simulink model "vcv_model"  (R2024b)
settings: Solver=VariableStepAuto  StartTime=0.0  StopTime=60.0  RelTol=1e-3
values from neighbouring files (symbols this model uses):
  C = 0.0965    [vcv.m]
  R = 4    [vcv.m]
libraries: slpidlib x2
settings Model: Creator=Neuer Benutzer  LastModifiedBy=Neuer Benutzer

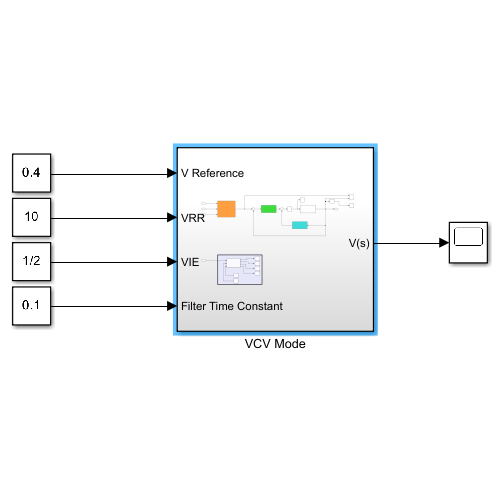
[thumbnail: Simulink's stored preview of the top-level diagram]
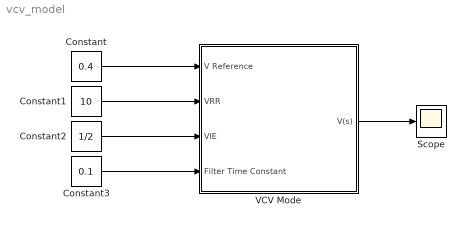
== system vcv_model ==
  Constant : Constant  Value=0.4
  Constant1 : Constant  Value=10
  Constant2 : Constant  Value=1/2
  Constant3 : Constant  Value=0.1
  Scope : Scope
  VCV Mode : Subsystem
  wires:
  Constant/1 -> VCV Mode/1(V Reference)
  Constant1/1 -> VCV Mode/2("VRR ")
  Constant2/1 -> VCV Mode/3(VIE)
  Constant3/1 -> VCV Mode/4("Filter Time Constant ")
  VCV Mode/1(V(s)) -> Scope/1

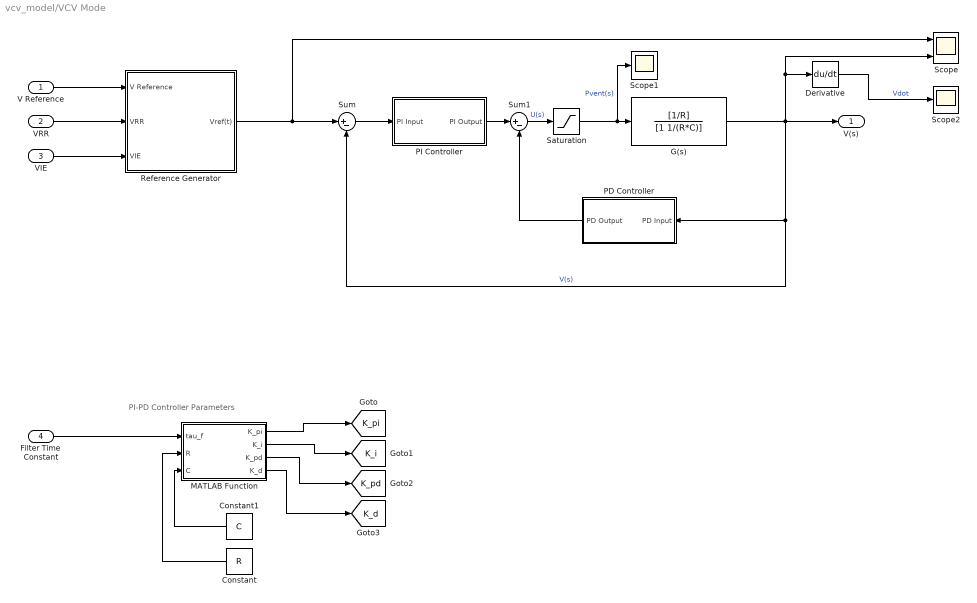
== system vcv_model/VCV Mode ==
  note: PI-PD Controller Parameters
  V Reference : Inport
  "VRR " : Inport  Port=2
  VIE : Inport  Port=3
  "Filter Time Constant " : Inport  Port=4
  Constant : Constant  Value=R
  Constant1 : Constant  Value=C
  Derivative : Derivative
  G(s) : TransferFcn  Numerator=[1/R]  Denominator=[1 1/(R*C)]
  MATLAB Function : MATLAB Function  TreatAsAtomicUnit=on
  PD Controller : Subsystem
  PI Controller : Subsystem
  Reference Generator : Subsystem
  Saturation : Saturate  UpperLimit=30  LowerLimit=0
  Scope : Scope  NumInputPorts=2
  Scope1 : Scope
  Scope2 : Scope
  Sum : Sum  Inputs=|+-
  Sum1 : Sum  Inputs=|+-
  V(s) : Outport
  tag scope: K_d=global, K_i=global, K_pd=global, K_pi=global
  wires:
  G(s)/1 -> Derivative/1, Scope/2, V(s)/1, Sum/2, PD Controller/1(PD Input)  "V(s)"
  Reference Generator/1(Vref(t)) -> Sum/1, Scope/1
  Saturation/1 -> Scope1/1, G(s)/1  "Pvent(s)"
  PD Controller/1(PD Output) -> Sum1/2
  "Filter Time Constant "/1 -> MATLAB Function/1(tau_f)
  "VRR "/1 -> Reference Generator/2("VRR ")
  V Reference/1 -> Reference Generator/1(V Reference)
  VIE/1 -> Reference Generator/3(VIE)
  PI Controller/1(PI Output) -> Sum1/1
  Sum/1 -> PI Controller/1(PI Input)
  Sum1/1 -> Saturation/1  "U(s)"
  MATLAB Function/1(K_pi) -> [K_pi]
  MATLAB Function/2(K_i) -> [K_i]
  MATLAB Function/3(K_pd) -> [K_pd]
  MATLAB Function/4(K_d) -> [K_d]
  Constant/1 -> MATLAB Function/2(R)
  Constant1/1 -> MATLAB Function/3(C)
  Derivative/1 -> Scope2/1  "Vdot"

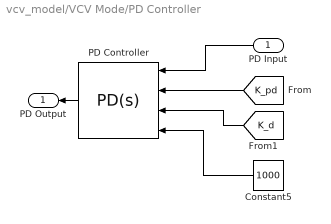
== system vcv_model/VCV Mode/PD Controller ==
  PD Input : Inport
  Constant5 : Constant  Value=1000
  PD Controller : slpidlib/PID Controller  Controller=PD  Form=Parallel  TimeDomain=Continuous-time  UseExternalTs=off  SampleTime=-1  IntegratorMethod=Forward Euler  FilterMethod=Forward Euler  ControllerParametersSource=external  P=1  I=1  UseKiTs=off  D=0  UseExternalDerivativeSource=off  N=100  UseFilter=on  TunerSelectOption=Transfer Function Based (PID Tuner App)  InitialConditionSource=internal  InitialConditionForIntegrator=0  InitialConditionForFilter=0  DifferentiatorICPrevScaledInput=0  ExternalReset=none  TrackingMode=off  Kt=1  LimitOutput=off  SatLimitsSource=internal  UpperSaturationLimit=30  LowerSaturationLimit=0  LinearizeAsGain=on  AntiWindupMode=none  Kb=1  LimitIntegrator=off  UpperIntegratorSaturationLimit=inf  LowerIntegratorSaturationLimit=-inf  POutMin=[]  POutMax=[]  IOutMin=[]  IOutMax=[]  DOutMin=[]  DOutMax=[]  NOutMin=[]  NOutMax=[]  SumOutMin=[]  SumOutMax=[]  SaturationOutMin=[]  SaturationOutMax=[]  PParamMin=[]  PParamMax=[]  IParamMin=[]  IParamMax=[]  DParamMin=[]  DParamMax=[]  NParamMin=[]  NParamMax=[]  KbParamMin=[]  KbParamMax=[]  KtParamMin=[]  KtParamMax=[]  KbOutMin=[]  KbOutMax=[]  KtOutMin=[]  KtOutMax=[]  IntegratorOutMin=[]  IntegratorOutMax=[]  FilterOutMin=[]  FilterOutMax=[]  SumI1OutMin=[]  SumI1OutMax=[]  SumI2OutMin=[]  SumI2OutMax=[]  SumI3OutMin=[]  SumI3OutMax=[]  SumI4OutMin=[]  SumI4OutMax=[]  SumDOutMin=[]  SumDOutMax=[]  DifferentiatorOutMin=[]  DifferentiatorOutMax=[]  FilterDiffOutCoefMin=[]  FilterDiffOutCoefMax=[]  ReciprocalOutMin=[]  ReciprocalOutMax=[]  SumDenOutMin=[]  SumDenOutMax=[]  SumNumOutMin=[]  SumNumOutMax=[]  DivideOutMin=[]  DivideOutMax=[]  UdiffTsProdOutMin=[]  UdiffTsProdOutMax=[]  NTsProdOutMin=[]  NTsProdOutMax=[]  UintegralTsProdOutMin=[]  UintegralTsProdOutMax=[]  UngainTsProdOutMin=[]  UngainTsProdOutMax=[]  ClampingZeroOutDataTypeStr=Inherit: Inherit via back propagation  ClampingZeroOutMin=[]  ClampingZeroOutMax=[]  FilterDenConstantOutDataTypeStr=Inherit: Inherit via back propagation  FilterDenConstantOutMin=[]  FilterDenConstantOutMax=[]  PCopyOutDataTypeStr=Inherit: Inherit via back propagation  PCopyOutMin=[]  PCopyOutMax=[]  NCopyOutDataTypeStr=Inherit: Inherit via back propagation  NCopyOutMin=[]  NCopyOutMax=[]  IntegratorContinuousStateAttributes=''  IntegratorStateMustResolveToSignalObject=off  IntegratorRTWStateStorageClass=Auto  FilterContinuousStateAttributes=''  FilterStateMustResolveToSignalObject=off  FilterRTWStateStorageClass=Auto  ParallelPVariant=ExternalParameters  IdealPVariant=Disabled  IVariant=Disabled  DVariant=ExternalParameters  IntegratorVariant=Disabled  SatVariant=Disabled  AWVariant=Disabled  PCopyVariant=Disabled  TRVariant=Disabled  FdbkBlocksVariant=Forward  IdealPFdbkVariant=Disabled  SatFdbkVariant=Disabled  DerivativeFilterVariant=ContFilter  NVariant=ExternalParameters  NCopyVariant=Disabled  FilterICVariant=InternalICsFilter  IntegratorICVariant=Disabled  ExternalResetVariant=Disabled  TRSumVariant=Passthrough  SumFdbkVariant=Disabled  SumVariant=Sum_PD  TsampFilterVariant=InternalTs  TsampNgainVariant=Passthrough  TsampIntegralVariant=Disabled_SignalSpec  ExternalSaturationOutDataTypeStr=Inherit: Same as second input  DerivativeSourceVariant=ErrorSignal  PreIntVariant=InternalPreInt
      settings: LibrarySourceBlock=cstblocks/Linear Parameter Varying/Varying PID Controller
  PD Output : Outport
  wires:
  PD Controller/1 -> PD Output/1
  Constant5/1 -> PD Controller/4
  PD Input/1 -> PD Controller/1
  [K_pd] -> PD Controller/2
  [K_d] -> PD Controller/3

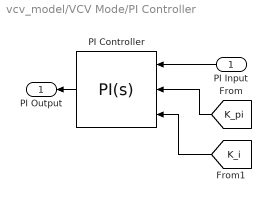
== system vcv_model/VCV Mode/PI Controller ==
  PI Input : Inport
  PI Controller : slpidlib/PID Controller  Controller=PI  Form=Parallel  TimeDomain=Continuous-time  UseExternalTs=off  SampleTime=-1  IntegratorMethod=Forward Euler  FilterMethod=Forward Euler  ControllerParametersSource=external  P=1  I=1  UseKiTs=off  D=0  UseExternalDerivativeSource=off  N=100  UseFilter=on  TunerSelectOption=Transfer Function Based (PID Tuner App)  InitialConditionSource=internal  InitialConditionForIntegrator=0  InitialConditionForFilter=0  DifferentiatorICPrevScaledInput=0  ExternalReset=none  TrackingMode=off  Kt=1  LimitOutput=off  SatLimitsSource=internal  UpperSaturationLimit=30  LowerSaturationLimit=0  LinearizeAsGain=on  AntiWindupMode=none  Kb=1  LimitIntegrator=off  UpperIntegratorSaturationLimit=inf  LowerIntegratorSaturationLimit=-inf  POutMin=[]  POutMax=[]  IOutMin=[]  IOutMax=[]  DOutMin=[]  DOutMax=[]  NOutMin=[]  NOutMax=[]  SumOutMin=[]  SumOutMax=[]  SaturationOutMin=[]  SaturationOutMax=[]  PParamMin=[]  PParamMax=[]  IParamMin=[]  IParamMax=[]  DParamMin=[]  DParamMax=[]  NParamMin=[]  NParamMax=[]  KbParamMin=[]  KbParamMax=[]  KtParamMin=[]  KtParamMax=[]  KbOutMin=[]  KbOutMax=[]  KtOutMin=[]  KtOutMax=[]  IntegratorOutMin=[]  IntegratorOutMax=[]  FilterOutMin=[]  FilterOutMax=[]  SumI1OutMin=[]  SumI1OutMax=[]  SumI2OutMin=[]  SumI2OutMax=[]  SumI3OutMin=[]  SumI3OutMax=[]  SumI4OutMin=[]  SumI4OutMax=[]  SumDOutMin=[]  SumDOutMax=[]  DifferentiatorOutMin=[]  DifferentiatorOutMax=[]  FilterDiffOutCoefMin=[]  FilterDiffOutCoefMax=[]  ReciprocalOutMin=[]  ReciprocalOutMax=[]  SumDenOutMin=[]  SumDenOutMax=[]  SumNumOutMin=[]  SumNumOutMax=[]  DivideOutMin=[]  DivideOutMax=[]  UdiffTsProdOutMin=[]  UdiffTsProdOutMax=[]  NTsProdOutMin=[]  NTsProdOutMax=[]  UintegralTsProdOutMin=[]  UintegralTsProdOutMax=[]  UngainTsProdOutMin=[]  UngainTsProdOutMax=[]  ClampingZeroOutDataTypeStr=Inherit: Inherit via back propagation  ClampingZeroOutMin=[]  ClampingZeroOutMax=[]  FilterDenConstantOutDataTypeStr=Inherit: Inherit via back propagation  FilterDenConstantOutMin=[]  FilterDenConstantOutMax=[]  PCopyOutDataTypeStr=Inherit: Inherit via back propagation  PCopyOutMin=[]  PCopyOutMax=[]  NCopyOutDataTypeStr=Inherit: Inherit via back propagation  NCopyOutMin=[]  NCopyOutMax=[]  IntegratorContinuousStateAttributes=''  IntegratorStateMustResolveToSignalObject=off  IntegratorRTWStateStorageClass=Auto  FilterContinuousStateAttributes=''  FilterStateMustResolveToSignalObject=off  FilterRTWStateStorageClass=Auto  ParallelPVariant=ExternalParameters  IdealPVariant=Disabled  IVariant=ExternalParameters  DVariant=Disabled  IntegratorVariant=Continuous  SatVariant=Disabled  AWVariant=Passthrough  PCopyVariant=Disabled  TRVariant=Disabled  FdbkBlocksVariant=Forward  IdealPFdbkVariant=Disabled  SatFdbkVariant=Disabled  DerivativeFilterVariant=Disabled  NVariant=Disabled  NCopyVariant=Disabled_SignalSpec  FilterICVariant=Disabled  IntegratorICVariant=InternalICs  ExternalResetVariant=Disabled  TRSumVariant=Passthrough  SumFdbkVariant=Disabled  SumVariant=Sum_PI  TsampFilterVariant=InternalTs  TsampNgainVariant=Passthrough  TsampIntegralVariant=Disabled_SignalSpec  ExternalSaturationOutDataTypeStr=Inherit: Same as second input  DerivativeSourceVariant=Disabled  PreIntVariant=InternalPreInt
      settings: LibrarySourceBlock=cstblocks/Linear Parameter Varying/Varying PID Controller
  PI Output : Outport
  wires:
  PI Input/1 -> PI Controller/1
  PI Controller/1 -> PI Output/1
  [K_pi] -> PI Controller/2
  [K_i] -> PI Controller/3

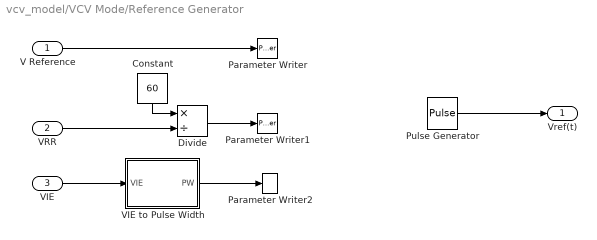
== system vcv_model/VCV Mode/Reference Generator ==
  V Reference : Inport
  "VRR " : Inport  Port=2
  VIE : Inport  Port=3
  Constant : Constant  Value=60
  Divide : Product  Inputs=*/
  Parameter Writer : ParameterWriter  ParameterOwnerBlock=../Pulse Generator  ParameterName=Amplitude  ParameterInternalName=Amplitude
  Parameter Writer1 : ParameterWriter  ParameterOwnerBlock=../Pulse Generator  ParameterName=Period  ParameterInternalName=Period
  Parameter Writer2 : ParameterWriter  ParameterOwnerBlock=../Pulse Generator  ParameterName=PulseWidth  ParameterInternalName=PulseWidth
  Pulse Generator : DiscretePulseGenerator  PulseType=Time based  Amplitude=10  Period=1  PulseWidth=70
  VIE to Pulse Width : MATLAB Function  TreatAsAtomicUnit=on
  Vref(t) : Outport
  wires:
  Constant/1 -> Divide/1
  Pulse Generator/1 -> Vref(t)/1
  "VRR "/1 -> Divide/2
  Divide/1 -> Parameter Writer1/1
  VIE/1 -> VIE to Pulse Width/1(VIE)
  V Reference/1 -> Parameter Writer/1
  VIE to Pulse Width/1(PW) -> Parameter Writer2/1

== matlab function vcv_model/VCV Mode/MATLAB Function ==
  data: tau_f input; K_pi output; K_i output; K_pd output; K_d output; R input; C input
function [K_pi, K_i, K_pd, K_d] = params(tau_f, R, C)

K_pi = (16 * R) / (25 * tau_f);
K_i  = (64 * R) / (25 * tau_f^2);
K_pd = (32 * R) / (5 * tau_f) - (1 / C);
K_d  = (23 * R) / 5 - (tau_f / C);

end

== matlab function vcv_model/VCV Mode/Reference Generator/VIE to Pulse Width ==
  data: VIE input; PW output
function PW = toPW(VIE)
 
PW = 100 * VIE / (1 + VIE);
